simulink model "Project1_SPXMMA001"  (R2021a)
settings: Solver=ode1  StartTime=0.0  StopTime=Inf  RelTol=1e-3
InitFcn:
  |  TOFF_InitialValue.PRE = 12000;
  | OFF_InitialValue.PRE = 12000;
  | TON_InitialValue.PRE = 2000;
  | ON_InitialValue.PRE = 2000;
  | T2OFF_InitialValue.PRE = 11000;
  | T2ON_InitialValue.PRE = 3000;
  | T3OFF_InitialValue.PRE = 5000;
undefined symbols (not defined in the file): BOOL, DINT, slplc
libraries: simulink x7
(part 2 of 13)

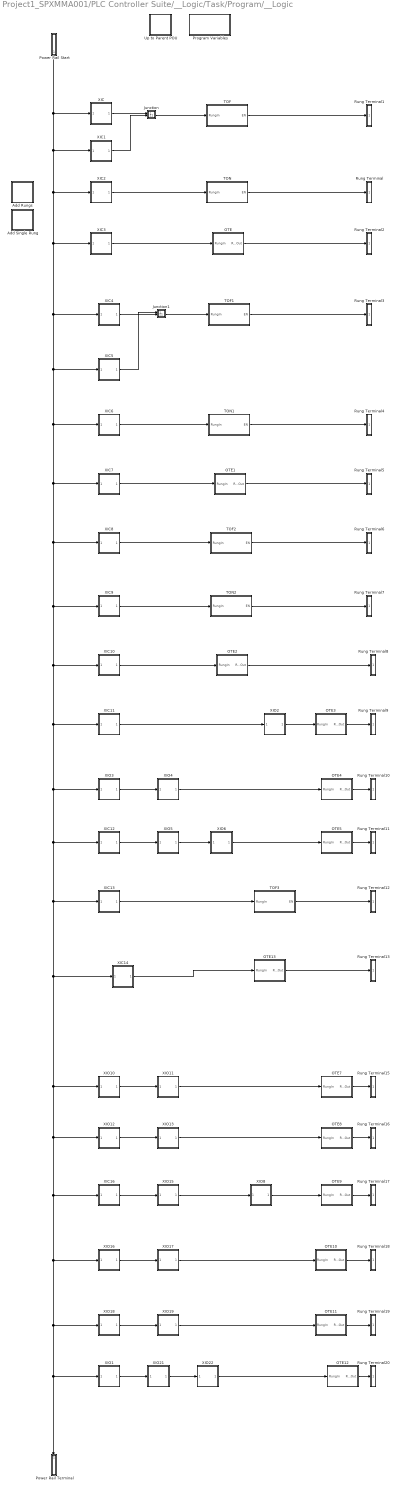
== system Project1_SPXMMA001/PLC Controller Suite/__Logic/Task/Program/__Logic ==
  Add Rungs : Subsystem  DisableCoverage=on  TreatAsAtomicUnit=on  mask{PLCRungNumberToAdd=2, PLCBlockType=AddRungs}
      mask prompts: PLCRungNumberToAdd "Rung Number:"
      mask Help: web([docroot '/plccoder/ref/addrungs' '.html']);
      mask DialogControl PLCAddRungs Prompt: Add Rungs
      mask DialogControl PLCRungAddButton Prompt: Add
      mask DialogControl PLCRungAddButton Callback: slplc.callbacks.addLadderRungs(gcb);
      mask Display: disp(sprintf(['Add' newline 'Rungs']));
  Add Single Rung : Subsystem  DisableCoverage=on  TreatAsAtomicUnit=on  mask{PLCRungNumberToAdd=1, PLCBlockType=AddSingleRung}
      settings: OpenFcn=slplc.callbacks.addLadderRungs(gcb);
      mask Help: web([docroot '/plccoder/ref/addsinglerung' '.html']);
      mask DialogControl PLCAddRung Prompt: Add Single Rung
      mask Display: disp(sprintf(['Add' newline '1 Rung']));
  Junction : Subsystem  Priority=4  DisableCoverage=on  TreatAsAtomicUnit=on  mask{PLCBlockType=Junction, PLCPOUType=BranchJunction}
      mask Help: web([docroot '/plccoder/ref/junction' '.html']);
      mask DialogControl PLCBlockTitle Prompt: Rung Merge Point
      mask DialogControl PLCBlockDesc Prompt: This is the ladder diagram rung merge point.
  Junction1 : Subsystem  Priority=15  DisableCoverage=on  TreatAsAtomicUnit=on  mask{PLCBlockType=Junction, PLCPOUType=BranchJunction}
      mask Help: web([docroot '/plccoder/ref/junction' '.html']);
      mask DialogControl PLCBlockTitle Prompt: Rung Merge Point
      mask DialogControl PLCBlockDesc Prompt: This is the ladder diagram rung merge point.
  OTE : Subsystem  Priority=11  TreatAsAtomicUnit=on  mask{PLCOperandTag=PED1_CROSS, PLCBlockType=OTE, PLCPOUType=Coil, PLCOperandExpression=xxx_PLC_VAR_PED1_CROSS}
      mask prompts: PLCOperandTag "Operand Tag:"
      mask init:
      | slplc.callbacks.initInstruction(gcb);
      settings: AttributesFormatString=%<PLCOperandTag>
      mask Help: web([docroot '/plccoder/ref/ote' '.html']);
      mask DialogControl PLCBlockTitle Prompt: Output Energize (OTE)
  OTE1 : Subsystem  Priority=22  TreatAsAtomicUnit=on  mask{PLCOperandTag=PED2_CROSS, PLCBlockType=OTE, PLCPOUType=Coil, PLCOperandExpression=xxx_PLC_VAR_PED2_CROSS}
      mask prompts: PLCOperandTag "Operand Tag:"
      mask init:
      | slplc.callbacks.initInstruction(gcb);
      settings: AttributesFormatString=%<PLCOperandTag>
      mask Help: web([docroot '/plccoder/ref/ote' '.html']);
      mask DialogControl PLCBlockTitle Prompt: Output Energize (OTE)
  OTE10 : Subsystem  Priority=67  TreatAsAtomicUnit=on  mask{PLCOperandTag=TL1_STOP, PLCBlockType=OTE, PLCPOUType=Coil, PLCOperandExpression=xxx_PLC_VAR_TL1_STOP}
      mask prompts: PLCOperandTag "Operand Tag:"
      mask init:
      | slplc.callbacks.initInstruction(gcb);
      settings: AttributesFormatString=%<PLCOperandTag>
      mask Help: web([docroot '/plccoder/ref/ote' '.html']);
      mask DialogControl PLCBlockTitle Prompt: Output Energize (OTE)
  OTE11 : Subsystem  Priority=71  TreatAsAtomicUnit=on  mask{PLCOperandTag=TL1_SO, PLCBlockType=OTE, PLCPOUType=Coil, PLCOperandExpression=xxx_PLC_VAR_TL1_SO}
      mask prompts: PLCOperandTag "Operand Tag:"
      mask init:
      | slplc.callbacks.initInstruction(gcb);
      settings: AttributesFormatString=%<PLCOperandTag>
      mask Help: web([docroot '/plccoder/ref/ote' '.html']);
      mask DialogControl PLCBlockTitle Prompt: Output Energize (OTE)
  OTE12 : Subsystem  Priority=76  TreatAsAtomicUnit=on  mask{PLCOperandTag=TL1_RO, PLCBlockType=OTE, PLCPOUType=Coil, PLCOperandExpression=xxx_PLC_VAR_TL1_RO}
      mask prompts: PLCOperandTag "Operand Tag:"
      mask init:
      | slplc.callbacks.initInstruction(gcb);
      settings: AttributesFormatString=%<PLCOperandTag>
      mask Help: web([docroot '/plccoder/ref/ote' '.html']);
      mask DialogControl PLCBlockTitle Prompt: Output Energize (OTE)
  OTE13 : Subsystem  Priority=50  TreatAsAtomicUnit=on  mask{PLCOperandTag=ZONE2_SENSOR, PLCBlockType=OTE, PLCPOUType=Coil, PLCOperandExpression=xxx_PLC_VAR_ZONE2_SENSOR}
      mask prompts: PLCOperandTag "Operand Tag:"
      mask init:
      | slplc.callbacks.initInstruction(gcb);
      settings: AttributesFormatString=%<PLCOperandTag>
      mask Help: web([docroot '/plccoder/ref/ote' '.html']);
      mask DialogControl PLCBlockTitle Prompt: Output Energize (OTE)
  OTE2 : Subsystem  Priority=31  TreatAsAtomicUnit=on  mask{PLCOperandTag=ZONE1_SENSOR, PLCBlockType=OTE, PLCPOUType=Coil, PLCOperandExpression=xxx_PLC_VAR_ZONE1_SENSOR}
      mask prompts: PLCOperandTag "Operand Tag:"
      mask init:
      | slplc.callbacks.initInstruction(gcb);
      settings: AttributesFormatString=%<PLCOperandTag>
      mask Help: web([docroot '/plccoder/ref/ote' '.html']);
      mask DialogControl PLCBlockTitle Prompt: Output Energize (OTE)
  OTE3 : Subsystem  Priority=35  TreatAsAtomicUnit=on  mask{PLCOperandTag=TL3_RO, PLCBlockType=OTE, PLCPOUType=Coil, PLCOperandExpression=xxx_PLC_VAR_TL3_RO}
      mask prompts: PLCOperandTag "Operand Tag:"
      mask init:
      | slplc.callbacks.initInstruction(gcb);
      settings: AttributesFormatString=%<PLCOperandTag>
      mask Help: web([docroot '/plccoder/ref/ote' '.html']);
      mask DialogControl PLCBlockTitle Prompt: Output Energize (OTE)
  OTE4 : Subsystem  Priority=39  TreatAsAtomicUnit=on  mask{PLCOperandTag=TL3_STOP, PLCBlockType=OTE, PLCPOUType=Coil, PLCOperandExpression=xxx_PLC_VAR_TL3_STOP}
      mask prompts: PLCOperandTag "Operand Tag:"
      mask init:
      | slplc.callbacks.initInstruction(gcb);
      settings: AttributesFormatString=%<PLCOperandTag>
      mask Help: web([docroot '/plccoder/ref/ote' '.html']);
      mask DialogControl PLCBlockTitle Prompt: Output Energize (OTE)
  OTE5 : Subsystem  Priority=44  TreatAsAtomicUnit=on  mask{PLCOperandTag=TL3_LO, PLCBlockType=OTE, PLCPOUType=Coil, PLCOperandExpression=xxx_PLC_VAR_TL3_LO}
      mask prompts: PLCOperandTag "Operand Tag:"
      mask init:
      | slplc.callbacks.initInstruction(gcb);
      settings: AttributesFormatString=%<PLCOperandTag>
      mask Help: web([docroot '/plccoder/ref/ote' '.html']);
      mask DialogControl PLCBlockTitle Prompt: Output Energize (OTE)
  OTE7 : Subsystem  Priority=54  TreatAsAtomicUnit=on  mask{PLCOperandTag=TL2_STOP, PLCBlockType=OTE, PLCPOUType=Coil, PLCOperandExpression=xxx_PLC_VAR_TL2_STOP}
      mask prompts: PLCOperandTag "Operand Tag:"
      mask init:
      | slplc.callbacks.initInstruction(gcb);
      settings: AttributesFormatString=%<PLCOperandTag>
      mask Help: web([docroot '/plccoder/ref/ote' '.html']);
      mask DialogControl PLCBlockTitle Prompt: Output Energize (OTE)
  OTE8 : Subsystem  Priority=58  TreatAsAtomicUnit=on  mask{PLCOperandTag=TL2_LO, PLCBlockType=OTE, PLCPOUType=Coil, PLCOperandExpression=xxx_PLC_VAR_TL2_LO}
      mask prompts: PLCOperandTag "Operand Tag:"
      mask init:
      | slplc.callbacks.initInstruction(gcb);
      settings: AttributesFormatString=%<PLCOperandTag>
      mask Help: web([docroot '/plccoder/ref/ote' '.html']);
      mask DialogControl PLCBlockTitle Prompt: Output Energize (OTE)
  OTE9 : Subsystem  Priority=63  TreatAsAtomicUnit=on  mask{PLCOperandTag=TL2_SO, PLCBlockType=OTE, PLCPOUType=Coil, PLCOperandExpression=xxx_PLC_VAR_TL2_SO}
      mask prompts: PLCOperandTag "Operand Tag:"
      mask init:
      | slplc.callbacks.initInstruction(gcb);
      settings: AttributesFormatString=%<PLCOperandTag>
      mask Help: web([docroot '/plccoder/ref/ote' '.html']);
      mask DialogControl PLCBlockTitle Prompt: Output Energize (OTE)
  Power Rail Start : Subsystem  Priority=1  DisableCoverage=on  TreatAsAtomicUnit=on  mask{PLCBlockType=PowerRailStart}
      mask Help: web([docroot '/plccoder/ref/powerrailstart' '.html']);
      mask DialogControl PLCBlockTitle Prompt: Power Rail Start
      mask DialogControl PLCBlockDesc Prompt: This is the ladder diagram left power rail start block.
  Power Rail Terminal : Subsystem  DisableCoverage=on  TreatAsAtomicUnit=on  mask{PLCBlockType=PowerRailTerminal}
      mask Help: web([docroot '/plccoder/ref/powerrailterminal' '.html']);
      mask DialogControl PLCBlockTitle Prompt: Power Rail Terminal
      mask DialogControl PLCBlockDesc Prompt: This is the ladder diagram left power rail terminal block.
  Program Variables : Subsystem  Tag=ProgramVariableSS  DisableCoverage=on  TreatAsAtomicUnit=on  mask{PLCVarOFFName=OFF, PLCVarOFFScope=Local, PLCVarOFFPortType=Hidden, PLCVarOFFPortIndex=32, PLCVarOFFDataType=Bus: TIMER, PLCVarOFFSize=1, PLCVarOFFInitialValue=OFF_InitialValue, PLCVarOFFToDelete=off, PLCVarONName=ON, PLCVarONScope=Local, PLCVarONPortType=Hidden, PLCVarONPortIndex=32, PLCVarONDataType=Bus: TIMER, PLCVarONSize=1, PLCVarONInitialValue=ON_InitialValue, PLCVarONToDelete=off, PLCVarPED1Name=PED1, PLCVarPED1Scope=Local, PLCVarPED1PortType=Hidden, PLCVarPED1PortIndex=32, PLCVarPED1DataType=BOOL, PLCVarPED1Size=1, PLCVarPED1InitialValue=false, PLCVarPED1ToDelete=off, PLCVarPED2Name=PED2, PLCVarPED2Scope=Local, PLCVarPED2PortType=Hidden, PLCVarPED2PortIndex=32, PLCVarPED2DataType=boolean, PLCVarPED2Size=1, PLCVarPED2InitialValue=false, PLCVarPED2ToDelete=off, PLCVarPED_CROSSName=PED_CROSS, PLCVarPED_CROSSScope=Local, PLCVarPED_CROSSPortType=Hidden, PLCVarPED_CROSSPortIndex=32, PLCVarPED_CROSSDataType=BOOL, PLCVarPED_CROSSSize=1, PLCVarPED_CROSSInitialValue=false, PLCVarPED_CROSSToDelete=off, PLCVarT2OFFName=T2OFF, PLCVarT2OFFScope=Local, PLCVarT2OFFPortType=Hidden, PLCVarT2OFFPortIndex=32, PLCVarT2OFFDataType=Bus: TIMER, PLCVarT2OFFSize=1, PLCVarT2OFFInitialValue=T2OFF_InitialValue, PLCVarT2OFFToDelete=off, PLCVarT2ONName=T2ON, PLCVarT2ONScope=Local, PLCVarT2ONPortType=Hidden, PLCVarT2ONPortIndex=32, PLCVarT2ONDataType=Bus: TIMER, PLCVarT2ONSize=1, PLCVarT2ONInitialValue=T2ON_InitialValue, PLCVarT2ONToDelete=off, PLCVarT3OFFName=T3OFF, PLCVarT3OFFScope=Local, PLCVarT3OFFPortType=Hidden, PLCVarT3OFFPortIndex=32, PLCVarT3OFFDataType=Bus: TIMER, PLCVarT3OFFSize=1, PLCVarT3OFFInitialValue=TOF_InitialValue, PLCVarT3OFFToDelete=off, PLCVarT3ONName=T3ON, PLCVarT3ONScope=Local, PLCVarT3ONPortType=Hidden, PLCVarT3ONPortIndex=32, PLCVarT3ONDataType=Bus: TIMER, PLCVarT3ONSize=1, PLCVarT3ONInitialValue=TON_InitialValue, PLCVarT3ONToDelete=off, PLCVarTL1_NOName=TL1_NO, PLCVarTL1_NOScope=Local, PLCVarTL1_NOPortType=Hidden, PLCVarTL1_NOPortIndex=32, PLCVarTL1_NODataType=BOOL, PLCVarTL1_NOSize=1, PLCVarTL1_NOInitialValue=false, PLCVarTL1_NOToDelete=off, PLCVarTL2_NOName=TL2_NO, PLCVarTL2_NOScope=Local, PLCVarTL2_NOPortType=Hidden, PLCVarTL2_NOPortIndex=32, PLCVarTL2_NODataType=BOOL, PLCVarTL2_NOSize=1, PLCVarTL2_NOInitialValue=false, PLCVarTL2_NOToDelete=off, PLCVarTOFFName=TOFF, PLCVarTOFFScope=Local, PLCVarTOFFPortType=Hidden, PLCVarTOFFPortIndex=32, PLCVarTOFFDataType=Bus: TIMER, PLCVarTOFFSize=1, PLCVarTOFFInitialValue=TOFF_InitialValue, PLCVarTOFFToDelete=off, PLCVarTONName=TON, PLCVarTONScope=Local, PLCVarTONPortType=Hidden, PLCVarTONPortIndex=32, PLCVarTONDataType=Bus: TIMER, PLCVarTONSize=1, PLCVarTONInitialValue=TON_InitialValue, PLCVarTONToDelete=off, PLCVarZONE1_SENSORName=ZONE1_SENSOR, PLCVarZONE1_SENSORScope=Local, PLCVarZONE1_SENSORPortType=Hidden, PLCVarZONE1_SENSORPortIndex=32, PLCVarZONE1_SENSORDataType=BOOL, PLCVarZONE1_SENSORSize=1, PLCVarZONE1_SENSORInitialValue=false, PLCVarZONE1_SENSORToDelete=off, PLCVarZONE2_SENSORName=ZONE2_SENSOR, PLCVarZONE2_SENSORScope=Local, PLCVarZONE2_SENSORPortType=Hidden, PLCVarZONE2_SENSORPortIndex=32, PLCVarZONE2_SENSORDataType=BOOL, PLCVarZONE2_SENSORSize=1, PLCVarZONE2_SENSORInitialValue=false, PLCVarZONE2_SENSORToDelete=off, PLCVarPED1_1Name=PED1_1, PLCVarPED1_1Scope=External, PLCVarPED1_1PortType=Hidden, PLCVarPED1_1PortIndex=32, PLCVarPED1_1DataType=DINT, PLCVarPED1_1Size=-1, PLCVarPED1_1InitialValue=0, PLCVarPED1_1ToDelete=off, PLCVarPED1_2Name=PED1_2, PLCVarPED1_2Scope=External, PLCVarPED1_2PortType=Hidden, PLCVarPED1_2PortIndex=32, PLCVarPED1_2DataType=DINT, PLCVarPED1_2Size=-1, PLCVarPED1_2InitialValue=0, PLCVarPED1_2ToDelete=off, PLCVarPED1_CROSSName=PED1_CROSS, PLCVarPED1_CROSSScope=External, PLCVarPED1_CROSSPortType=Hidden, PLCVarPED1_CROSSPortIndex=32, PLCVarPED1_CROSSDataType=DINT, PLCVarPED1_CROSSSize=-1, PLCVarPED1_CROSSInitialValue=0, PLCVarPED1_CROSSToDelete=off, PLCVarPED2_1Name=PED2_1, PLCVarPED2_1Scope=External, PLCVarPED2_1PortType=Hidden, PLCVarPED2_1PortIndex=32, PLCVarPED2_1DataType=DINT, PLCVarPED2_1Size=-1, PLCVarPED2_1InitialValue=0, PLCVarPED2_1ToDelete=off, PLCVarPED2_2Name=PED2_2, PLCVarPED2_2Scope=External, PLCVarPED2_2PortType=Hidden, PLCVarPED2_2PortIndex=32, PLCVarPED2_2DataType=DINT, PLCVarPED2_2Size=-1, PLCVarPED2_2InitialValue=0, PLCVarPED2_2ToDelete=off, PLCVarPED2_CROSSName=PED2_CROSS, PLCVarPED2_CROSSScope=External, PLCVarPED2_CROSSPortType=Hidden, PLCVarPED2_CROSSPortIndex=32, PLCVarPED2_CROSSDataType=DINT, PLCVarPED2_CROSSSize=-1, PLCVarPED2_CROSSInitialValue=0, PLCVarPED2_CROSSToDelete=off, PLCVarTL1_ROName=TL1_RO, PLCVarTL1_ROScope=External, PLCVarTL1_ROPortType=Hidden, PLCVarTL1_ROPortIndex=32, PLCVarTL1_RODataType=DINT, PLCVarTL1_ROSize=-1, PLCVarTL1_ROInitialValue=0, PLCVarTL1_ROToDelete=off, PLCVarTL1_SOName=TL1_SO, PLCVarTL1_SOScope=External, PLCVarTL1_SOPortType=Hidden, PLCVarTL1_SOPortIndex=32, PLCVarTL1_SODataType=DINT, PLCVarTL1_SOSize=-1, PLCVarTL1_SOInitialValue=0, PLCVarTL1_SOToDelete=off, PLCVarTL1_STOPName=TL1_STOP, PLCVarTL1_STOPScope=External, PLCVarTL1_STOPPortType=Hidden, PLCVarTL1_STOPPortIndex=32, PLCVarTL1_STOPDataType=DINT, PLCVarTL1_STOPSize=-1, PLCVarTL1_STOPInitialValue=0, PLCVarTL1_STOPToDelete=off, PLCVarTL2_LOName=TL2_LO, PLCVarTL2_LOScope=External, PLCVarTL2_LOPortType=Hidden, PLCVarTL2_LOPortIndex=32, PLCVarTL2_LODataType=DINT, PLCVarTL2_LOSize=-1, PLCVarTL2_LOInitialValue=0, PLCVarTL2_LOToDelete=off, PLCVarTL2_SOName=TL2_SO, PLCVarTL2_SOScope=External, PLCVarTL2_SOPortType=Hidden, PLCVarTL2_SOPortIndex=32, PLCVarTL2_SODataType=DINT, PLCVarTL2_SOSize=-1, PLCVarTL2_SOInitialValue=0, PLCVarTL2_SOToDelete=off, PLCVarTL2_STOPName=TL2_STOP, PLCVarTL2_STOPScope=External, PLCVarTL2_STOPPortType=Hidden, PLCVarTL2_STOPPortIndex=32, PLCVarTL2_STOPDataType=DINT, PLCVarTL2_STOPSize=-1, PLCVarTL2_STOPInitialValue=0, PLCVarTL2_STOPToDelete=off, PLCVarTL3_LOName=TL3_LO, PLCVarTL3_LOScope=External, PLCVarTL3_LOPortType=Hidden, PLCVarTL3_LOPortIndex=32, PLCVarTL3_LODataType=DINT, PLCVarTL3_LOSize=-1, PLCVarTL3_LOInitialValue=0, PLCVarTL3_LOToDelete=off, PLCVarTL3_ROName=TL3_RO, PLCVarTL3_ROScope=External, PLCVarTL3_ROPortType=Hidden, PLCVarTL3_ROPortIndex=32, PLCVarTL3_RODataType=DINT, PLCVarTL3_ROSize=-1, PLCVarTL3_ROInitialValue=0, PLCVarTL3_ROToDelete=off, PLCVarTL3_STOPName=TL3_STOP, PLCVarTL3_STOPScope=External, PLCVarTL3_STOPPortType=Hidden, PLCVarTL3_STOPPortIndex=32, PLCVarTL3_STOPDataType=DINT, PLCVarTL3_STOPSize=-1, PLCVarTL3_STOPInitialValue=0, PLCVarTL3_STOPToDelete=off, PLCVarZONE1Name=ZONE1, PLCVarZONE1Scope=External, PLCVarZONE1PortType=Hidden, PLCVarZONE1PortIndex=32, PLCVarZONE1DataType=DINT, PLCVarZONE1Size=-1, PLCVarZONE1InitialValue=0, PLCVarZONE1ToDelete=off, PLCVarZONE2Name=ZONE2, PLCVarZONE2Scope=External, PLCVarZONE2PortType=Hidden, PLCVarZONE2PortIndex=32, PLCVarZONE2DataType=DINT, PLCVarZONE2Size=-1, PLCVarZONE2InitialValue=0, PLCVarZONE2ToDelete=off}
      mask init:
      | slplc.callbacks.initPOUVarSS(gcb);
      settings: OpenFcn=slplc.callbacks.openProgramVariableSS(gcb);
      mask Help: web([docroot '/plccoder/ref/programvariables' '.html']);
      mask TypeOptions PLCVarOFFScope: Local | External
      mask Callback PLCVarOFFScope: slplc.callbacks.updatePOUVarSS(gcb);
      mask TypeOptions PLCVarOFFPortType: Hidden | Inport | Outport
      mask Callback PLCVarOFFPortType: slplc.callbacks.updatePOUVarSS(gcb);
      mask TypeOptions PLCVarOFFPortIndex: 1 | 2 | 3 | 4 | 5 | 6 | 7 | 8 | 9 | 10 | 11 | 12 | 13 | 14 | 15 | 16 | 17 | 18 | 19 | 20 | 21 | 22 | 23 | 24 | 25 | 26 | 27 | 28 | 29 | 30 | 31 | 32
      mask TypeOptions PLCVarONScope: Local | External
      mask Callback PLCVarONScope: slplc.callbacks.updatePOUVarSS(gcb);
      mask TypeOptions PLCVarONPortType: Hidden | Inport | Outport
      mask Callback PLCVarONPortType: slplc.callbacks.updatePOUVarSS(gcb);
      mask TypeOptions PLCVarONPortIndex: 1 | 2 | 3 | 4 | 5 | 6 | 7 | 8 | 9 | 10 | 11 | 12 | 13 | 14 | 15 | 16 | 17 | 18 | 19 | 20 | 21 | 22 | 23 | 24 | 25 | 26 | 27 | 28 | 29 | 30 | 31 | 32
      mask TypeOptions PLCVarPED1Scope: Local | External
      mask Callback PLCVarPED1Scope: slplc.callbacks.updatePOUVarSS(gcb);
      mask TypeOptions PLCVarPED1PortType: Hidden | Inport | Outport
      mask Callback PLCVarPED1PortType: slplc.callbacks.updatePOUVarSS(gcb);
      mask TypeOptions PLCVarPED1PortIndex: 1 | 2 | 3 | 4 | 5 | 6 | 7 | 8 | 9 | 10 | 11 | 12 | 13 | 14 | 15 | 16 | 17 | 18 | 19 | 20 | 21 | 22 | 23 | 24 | 25 | 26 | 27 | 28 | 29 | 30 | 31 | 32
      mask TypeOptions PLCVarPED2Scope: Local | External
      mask Callback PLCVarPED2Scope: slplc.callbacks.updatePOUVarSS(gcb);
      mask TypeOptions PLCVarPED2PortType: Hidden | Inport | Outport
      mask Callback PLCVarPED2PortType: slplc.callbacks.updatePOUVarSS(gcb);
      mask TypeOptions PLCVarPED2PortIndex: 1 | 2 | 3 | 4 | 5 | 6 | 7 | 8 | 9 | 10 | 11 | 12 | 13 | 14 | 15 | 16 | 17 | 18 | 19 | 20 | 21 | 22 | 23 | 24 | 25 | 26 | 27 | 28 | 29 | 30 | 31 | 32
      mask TypeOptions PLCVarPED_CROSSScope: Local | External
      mask Callback PLCVarPED_CROSSScope: slplc.callbacks.updatePOUVarSS(gcb);
      mask TypeOptions PLCVarPED_CROSSPortType: Hidden | Inport | Outport
      mask Callback PLCVarPED_CROSSPortType: slplc.callbacks.updatePOUVarSS(gcb);
      mask TypeOptions PLCVarPED_CROSSPortIndex: 1 | 2 | 3 | 4 | 5 | 6 | 7 | 8 | 9 | 10 | 11 | 12 | 13 | 14 | 15 | 16 | 17 | 18 | 19 | 20 | 21 | 22 | 23 | 24 | 25 | 26 | 27 | 28 | 29 | 30 | 31 | 32
      mask TypeOptions PLCVarT2OFFScope: Local | External
      mask Callback PLCVarT2OFFScope: slplc.callbacks.updatePOUVarSS(gcb);
      mask TypeOptions PLCVarT2OFFPortType: Hidden | Inport | Outport
      mask Callback PLCVarT2OFFPortType: slplc.callbacks.updatePOUVarSS(gcb);
      mask TypeOptions PLCVarT2OFFPortIndex: 1 | 2 | 3 | 4 | 5 | 6 | 7 | 8 | 9 | 10 | 11 | 12 | 13 | 14 | 15 | 16 | 17 | 18 | 19 | 20 | 21 | 22 | 23 | 24 | 25 | 26 | 27 | 28 | 29 | 30 | 31 | 32
      mask TypeOptions PLCVarT2ONScope: Local | External
      mask Callback PLCVarT2ONScope: slplc.callbacks.updatePOUVarSS(gcb);
      mask TypeOptions PLCVarT2ONPortType: Hidden | Inport | Outport
      mask Callback PLCVarT2ONPortType: slplc.callbacks.updatePOUVarSS(gcb);
      mask TypeOptions PLCVarT2ONPortIndex: 1 | 2 | 3 | 4 | 5 | 6 | 7 | 8 | 9 | 10 | 11 | 12 | 13 | 14 | 15 | 16 | 17 | 18 | 19 | 20 | 21 | 22 | 23 | 24 | 25 | 26 | 27 | 28 | 29 | 30 | 31 | 32
      mask TypeOptions PLCVarT3OFFScope: Local | External
      mask Callback PLCVarT3OFFScope: slplc.callbacks.updatePOUVarSS(gcb);
      mask TypeOptions PLCVarT3OFFPortType: Hidden | Inport | Outport
      mask Callback PLCVarT3OFFPortType: slplc.callbacks.updatePOUVarSS(gcb);
      mask TypeOptions PLCVarT3OFFPortIndex: 1 | 2 | 3 | 4 | 5 | 6 | 7 | 8 | 9 | 10 | 11 | 12 | 13 | 14 | 15 | 16 | 17 | 18 | 19 | 20 | 21 | 22 | 23 | 24 | 25 | 26 | 27 | 28 | 29 | 30 | 31 | 32
      mask TypeOptions PLCVarT3ONScope: Local | External
      mask Callback PLCVarT3ONScope: slplc.callbacks.updatePOUVarSS(gcb);
      mask TypeOptions PLCVarT3ONPortType: Hidden | Inport | Outport
      mask Callback PLCVarT3ONPortType: slplc.callbacks.updatePOUVarSS(gcb);
      mask TypeOptions PLCVarT3ONPortIndex: 1 | 2 | 3 | 4 | 5 | 6 | 7 | 8 | 9 | 10 | 11 | 12 | 13 | 14 | 15 | 16 | 17 | 18 | 19 | 20 | 21 | 22 | 23 | 24 | 25 | 26 | 27 | 28 | 29 | 30 | 31 | 32
      mask TypeOptions PLCVarTL1_NOScope: Local | External
      mask Callback PLCVarTL1_NOScope: slplc.callbacks.updatePOUVarSS(gcb);
      mask TypeOptions PLCVarTL1_NOPortType: Hidden | Inport | Outport
      mask Callback PLCVarTL1_NOPortType: slplc.callbacks.updatePOUVarSS(gcb);
      mask TypeOptions PLCVarTL1_NOPortIndex: 1 | 2 | 3 | 4 | 5 | 6 | 7 | 8 | 9 | 10 | 11 | 12 | 13 | 14 | 15 | 16 | 17 | 18 | 19 | 20 | 21 | 22 | 23 | 24 | 25 | 26 | 27 | 28 | 29 | 30 | 31 | 32
      mask TypeOptions PLCVarTL2_NOScope: Local | External
      mask Callback PLCVarTL2_NOScope: slplc.callbacks.updatePOUVarSS(gcb);
      mask TypeOptions PLCVarTL2_NOPortType: Hidden | Inport | Outport
      mask Callback PLCVarTL2_NOPortType: slplc.callbacks.updatePOUVarSS(gcb);
      mask TypeOptions PLCVarTL2_NOPortIndex: 1 | 2 | 3 | 4 | 5 | 6 | 7 | 8 | 9 | 10 | 11 | 12 | 13 | 14 | 15 | 16 | 17 | 18 | 19 | 20 | 21 | 22 | 23 | 24 | 25 | 26 | 27 | 28 | 29 | 30 | 31 | 32
      mask TypeOptions PLCVarTOFFScope: Local | External
      mask Callback PLCVarTOFFScope: slplc.callbacks.updatePOUVarSS(gcb);
      mask TypeOptions PLCVarTOFFPortType: Hidden | Inport | Outport
      mask Callback PLCVarTOFFPortType: slplc.callbacks.updatePOUVarSS(gcb);
      mask TypeOptions PLCVarTOFFPortIndex: 1 | 2 | 3 | 4 | 5 | 6 | 7 | 8 | 9 | 10 | 11 | 12 | 13 | 14 | 15 | 16 | 17 | 18 | 19 | 20 | 21 | 22 | 23 | 24 | 25 | 26 | 27 | 28 | 29 | 30 | 31 | 32
      mask TypeOptions PLCVarTONScope: Local | External
      mask Callback PLCVarTONScope: slplc.callbacks.updatePOUVarSS(gcb);
      mask TypeOptions PLCVarTONPortType: Hidden | Inport | Outport
      mask Callback PLCVarTONPortType: slplc.callbacks.updatePOUVarSS(gcb);
      mask TypeOptions PLCVarTONPortIndex: 1 | 2 | 3 | 4 | 5 | 6 | 7 | 8 | 9 | 10 | 11 | 12 | 13 | 14 | 15 | 16 | 17 | 18 | 19 | 20 | 21 | 22 | 23 | 24 | 25 | 26 | 27 | 28 | 29 | 30 | 31 | 32
      mask TypeOptions PLCVarZONE1_SENSORScope: Local | External
      mask Callback PLCVarZONE1_SENSORScope: slplc.callbacks.updatePOUVarSS(gcb);
      mask TypeOptions PLCVarZONE1_SENSORPortType: Hidden | Inport | Outport
      mask Callback PLCVarZONE1_SENSORPortType: slplc.callbacks.updatePOUVarSS(gcb);
      mask TypeOptions PLCVarZONE1_SENSORPortIndex: 1 | 2 | 3 | 4 | 5 | 6 | 7 | 8 | 9 | 10 | 11 | 12 | 13 | 14 | 15 | 16 | 17 | 18 | 19 | 20 | 21 | 22 | 23 | 24 | 25 | 26 | 27 | 28 | 29 | 30 | 31 | 32
      mask TypeOptions PLCVarZONE2_SENSORScope: Local | External
      mask Callback PLCVarZONE2_SENSORScope: slplc.callbacks.updatePOUVarSS(gcb);
      mask TypeOptions PLCVarZONE2_SENSORPortType: Hidden | Inport | Outport
      mask Callback PLCVarZONE2_SENSORPortType: slplc.callbacks.updatePOUVarSS(gcb);
      mask TypeOptions PLCVarZONE2_SENSORPortIndex: 1 | 2 | 3 | 4 | 5 | 6 | 7 | 8 | 9 | 10 | 11 | 12 | 13 | 14 | 15 | 16 | 17 | 18 | 19 | 20 | 21 | 22 | 23 | 24 | 25 | 26 | 27 | 28 | 29 | 30 | 31 | 32
      mask TypeOptions PLCVarPED1_1Scope: Local | External
      mask Callback PLCVarPED1_1Scope: slplc.callbacks.updatePOUVarSS(gcb);
      mask TypeOptions PLCVarPED1_1PortType: Hidden | Inport | Outport
      mask Callback PLCVarPED1_1PortType: slplc.callbacks.updatePOUVarSS(gcb);
      mask TypeOptions PLCVarPED1_1PortIndex: 1 | 2 | 3 | 4 | 5 | 6 | 7 | 8 | 9 | 10 | 11 | 12 | 13 | 14 | 15 | 16 | 17 | 18 | 19 | 20 | 21 | 22 | 23 | 24 | 25 | 26 | 27 | 28 | 29 | 30 | 31 | 32
      mask TypeOptions PLCVarPED1_2Scope: Local | External
      mask Callback PLCVarPED1_2Scope: slplc.callbacks.updatePOUVarSS(gcb);
      mask TypeOptions PLCVarPED1_2PortType: Hidden | Inport | Outport
      mask Callback PLCVarPED1_2PortType: slplc.callbacks.updatePOUVarSS(gcb);
      mask TypeOptions PLCVarPED1_2PortIndex: 1 | 2 | 3 | 4 | 5 | 6 | 7 | 8 | 9 | 10 | 11 | 12 | 13 | 14 | 15 | 16 | 17 | 18 | 19 | 20 | 21 | 22 | 23 | 24 | 25 | 26 | 27 | 28 | 29 | 30 | 31 | 32
      mask TypeOptions PLCVarPED1_CROSSScope: Local | External
      mask Callback PLCVarPED1_CROSSScope: slplc.callbacks.updatePOUVarSS(gcb);
      mask TypeOptions PLCVarPED1_CROSSPortType: Hidden | Inport | Outport
      mask Callback PLCVarPED1_CROSSPortType: slplc.callbacks.updatePOUVarSS(gcb);
      mask TypeOptions PLCVarPED1_CROSSPortIndex: 1 | 2 | 3 | 4 | 5 | 6 | 7 | 8 | 9 | 10 | 11 | 12 | 13 | 14 | 15 | 16 | 17 | 18 | 19 | 20 | 21 | 22 | 23 | 24 | 25 | 26 | 27 | 28 | 29 | 30 | 31 | 32
      mask TypeOptions PLCVarPED2_1Scope: Local | External
      mask Callback PLCVarPED2_1Scope: slplc.callbacks.updatePOUVarSS(gcb);
      mask TypeOptions PLCVarPED2_1PortType: Hidden | Inport | Outport
      mask Callback PLCVarPED2_1PortType: slplc.callbacks.updatePOUVarSS(gcb);
      mask TypeOptions PLCVarPED2_1PortIndex: 1 | 2 | 3 | 4 | 5 | 6 | 7 | 8 | 9 | 10 | 11 | 12 | 13 | 14 | 15 | 16 | 17 | 18 | 19 | 20 | 21 | 22 | 23 | 24 | 25 | 26 | 27 | 28 | 29 | 30 | 31 | 32
      mask TypeOptions PLCVarPED2_2Scope: Local | External
      mask Callback PLCVarPED2_2Scope: slplc.callbacks.updatePOUVarSS(gcb);
      mask TypeOptions PLCVarPED2_2PortType: Hidden | Inport | Outport
      mask Callback PLCVarPED2_2PortType: slplc.callbacks.updatePOUVarSS(gcb);
      mask TypeOptions PLCVarPED2_2PortIndex: 1 | 2 | 3 | 4 | 5 | 6 | 7 | 8 | 9 | 10 | 11 | 12 | 13 | 14 | 15 | 16 | 17 | 18 | 19 | 20 | 21 | 22 | 23 | 24 | 25 | 26 | 27 | 28 | 29 | 30 | 31 | 32
      mask TypeOptions PLCVarPED2_CROSSScope: Local | External
      mask Callback PLCVarPED2_CROSSScope: slplc.callbacks.updatePOUVarSS(gcb);
      mask TypeOptions PLCVarPED2_CROSSPortType: Hidden | Inport | Outport
      mask Callback PLCVarPED2_CROSSPortType: slplc.callbacks.updatePOUVarSS(gcb);
      mask TypeOptions PLCVarPED2_CROSSPortIndex: 1 | 2 | 3 | 4 | 5 | 6 | 7 | 8 | 9 | 10 | 11 | 12 | 13 | 14 | 15 | 16 | 17 | 18 | 19 | 20 | 21 | 22 | 23 | 24 | 25 | 26 | 27 | 28 | 29 | 30 | 31 | 32
      mask TypeOptions PLCVarTL1_ROScope: Local | External
      mask Callback PLCVarTL1_ROScope: slplc.callbacks.updatePOUVarSS(gcb);
      mask TypeOptions PLCVarTL1_ROPortType: Hidden | Inport | Outport
      mask Callback PLCVarTL1_ROPortType: slplc.callbacks.updatePOUVarSS(gcb);
      mask TypeOptions PLCVarTL1_ROPortIndex: 1 | 2 | 3 | 4 | 5 | 6 | 7 | 8 | 9 | 10 | 11 | 12 | 13 | 14 | 15 | 16 | 17 | 18 | 19 | 20 | 21 | 22 | 23 | 24 | 25 | 26 | 27 | 28 | 29 | 30 | 31 | 32
      mask TypeOptions PLCVarTL1_SOScope: Local | External
      mask Callback PLCVarTL1_SOScope: slplc.callbacks.updatePOUVarSS(gcb);
      mask TypeOptions PLCVarTL1_SOPortType: Hidden | Inport | Outport
      mask Callback PLCVarTL1_SOPortType: slplc.callbacks.updatePOUVarSS(gcb);
      mask TypeOptions PLCVarTL1_SOPortIndex: 1 | 2 | 3 | 4 | 5 | 6 | 7 | 8 | 9 | 10 | 11 | 12 | 13 | 14 | 15 | 16 | 17 | 18 | 19 | 20 | 21 | 22 | 23 | 24 | 25 | 26 | 27 | 28 | 29 | 30 | 31 | 32
      mask TypeOptions PLCVarTL1_STOPScope: Local | External
      mask Callback PLCVarTL1_STOPScope: slplc.callbacks.updatePOUVarSS(gcb);
      mask TypeOptions PLCVarTL1_STOPPortType: Hidden | Inport | Outport
      mask Callback PLCVarTL1_STOPPortType: slplc.callbacks.updatePOUVarSS(gcb);
      mask TypeOptions PLCVarTL1_STOPPortIndex: 1 | 2 | 3 | 4 | 5 | 6 | 7 | 8 | 9 | 10 | 11 | 12 | 13 | 14 | 15 | 16 | 17 | 18 | 19 | 20 | 21 | 22 | 23 | 24 | 25 | 26 | 27 | 28 | 29 | 30 | 31 | 32
      mask TypeOptions PLCVarTL2_LOScope: Local | External
      mask Callback PLCVarTL2_LOScope: slplc.callbacks.updatePOUVarSS(gcb);
      mask TypeOptions PLCVarTL2_LOPortType: Hidden | Inport | Outport
      mask Callback PLCVarTL2_LOPortType: slplc.callbacks.updatePOUVarSS(gcb);
      mask TypeOptions PLCVarTL2_LOPortIndex: 1 | 2 | 3 | 4 | 5 | 6 | 7 | 8 | 9 | 10 | 11 | 12 | 13 | 14 | 15 | 16 | 17 | 18 | 19 | 20 | 21 | 22 | 23 | 24 | 25 | 26 | 27 | 28 | 29 | 30 | 31 | 32
      mask TypeOptions PLCVarTL2_SOScope: Local | External
      mask Callback PLCVarTL2_SOScope: slplc.callbacks.updatePOUVarSS(gcb);
      mask TypeOptions PLCVarTL2_SOPortType: Hidden | Inport | Outport
      mask Callback PLCVarTL2_SOPortType: slplc.callbacks.updatePOUVarSS(gcb);
      mask TypeOptions PLCVarTL2_SOPortIndex: 1 | 2 | 3 | 4 | 5 | 6 | 7 | 8 | 9 | 10 | 11 | 12 | 13 | 14 | 15 | 16 | 17 | 18 | 19 | 20 | 21 | 22 | 23 | 24 | 25 | 26 | 27 | 28 | 29 | 30 | 31 | 32
      mask TypeOptions PLCVarTL2_STOPScope: Local | External
      mask Callback PLCVarTL2_STOPScope: slplc.callbacks.updatePOUVarSS(gcb);
      mask TypeOptions PLCVarTL2_STOPPortType: Hidden | Inport | Outport
      mask Callback PLCVarTL2_STOPPortType: slplc.callbacks.updatePOUVarSS(gcb);
      mask TypeOptions PLCVarTL2_STOPPortIndex: 1 | 2 | 3 | 4 | 5 | 6 | 7 | 8 | 9 | 10 | 11 | 12 | 13 | 14 | 15 | 16 | 17 | 18 | 19 | 20 | 21 | 22 | 23 | 24 | 25 | 26 | 27 | 28 | 29 | 30 | 31 | 32
      mask TypeOptions PLCVarTL3_LOScope: Local | External
      mask Callback PLCVarTL3_LOScope: slplc.callbacks.updatePOUVarSS(gcb);
      mask TypeOptions PLCVarTL3_LOPortType: Hidden | Inport | Outport
      mask Callback PLCVarTL3_LOPortType: slplc.callbacks.updatePOUVarSS(gcb);
      mask TypeOptions PLCVarTL3_LOPortIndex: 1 | 2 | 3 | 4 | 5 | 6 | 7 | 8 | 9 | 10 | 11 | 12 | 13 | 14 | 15 | 16 | 17 | 18 | 19 | 20 | 21 | 22 | 23 | 24 | 25 | 26 | 27 | 28 | 29 | 30 | 31 | 32
      mask TypeOptions PLCVarTL3_ROScope: Local | External
      mask Callback PLCVarTL3_ROScope: slplc.callbacks.updatePOUVarSS(gcb);
      mask TypeOptions PLCVarTL3_ROPortType: Hidden | Inport | Outport
      mask Callback PLCVarTL3_ROPortType: slplc.callbacks.updatePOUVarSS(gcb);
      mask TypeOptions PLCVarTL3_ROPortIndex: 1 | 2 | 3 | 4 | 5 | 6 | 7 | 8 | 9 | 10 | 11 | 12 | 13 | 14 | 15 | 16 | 17 | 18 | 19 | 20 | 21 | 22 | 23 | 24 | 25 | 26 | 27 | 28 | 29 | 30 | 31 | 32
      mask TypeOptions PLCVarTL3_STOPScope: Local | External
      mask Callback PLCVarTL3_STOPScope: slplc.callbacks.updatePOUVarSS(gcb);
      mask TypeOptions PLCVarTL3_STOPPortType: Hidden | Inport | Outport
      mask Callback PLCVarTL3_STOPPortType: slplc.callbacks.updatePOUVarSS(gcb);
      mask TypeOptions PLCVarTL3_STOPPortIndex: 1 | 2 | 3 | 4 | 5 | 6 | 7 | 8 | 9 | 10 | 11 | 12 | 13 | 14 | 15 | 16 | 17 | 18 | 19 | 20 | 21 | 22 | 23 | 24 | 25 | 26 | 27 | 28 | 29 | 30 | 31 | 32
      mask TypeOptions PLCVarZONE1Scope: Local | External
      mask Callback PLCVarZONE1Scope: slplc.callbacks.updatePOUVarSS(gcb);
      mask TypeOptions PLCVarZONE1PortType: Hidden | Inport | Outport
      mask Callback PLCVarZONE1PortType: slplc.callbacks.updatePOUVarSS(gcb);
      mask TypeOptions PLCVarZONE1PortIndex: 1 | 2 | 3 | 4 | 5 | 6 | 7 | 8 | 9 | 10 | 11 | 12 | 13 | 14 | 15 | 16 | 17 | 18 | 19 | 20 | 21 | 22 | 23 | 24 | 25 | 26 | 27 | 28 | 29 | 30 | 31 | 32
      mask TypeOptions PLCVarZONE2Scope: Local | External
      mask Callback PLCVarZONE2Scope: slplc.callbacks.updatePOUVarSS(gcb);
      mask TypeOptions PLCVarZONE2PortType: Hidden | Inport | Outport
      mask Callback PLCVarZONE2PortType: slplc.callbacks.updatePOUVarSS(gcb);
      mask TypeOptions PLCVarZONE2PortIndex: 1 | 2 | 3 | 4 | 5 | 6 | 7 | 8 | 9 | 10 | 11 | 12 | 13 | 14 | 15 | 16 | 17 | 18 | 19 | 20 | 21 | 22 | 23 | 24 | 25 | 26 | 27 | 28 | 29 | 30 | 31 | 32
      mask DialogControl PLCBlockTitle Prompt: Program Variable Spreadsheet
      mask DialogControl PLCVarListHeaderName Prompt: Name
      mask DialogControl PLCVarListHeaderScope Prompt: Scope
      mask DialogControl PLCVarListHeaderDataType Prompt: Data Type
      mask DialogControl PLCVarListHeaderSize Prompt: Size
      mask DialogControl PLCVarListHeaderInitialValue Prompt: Initial Value
      mask DialogControl PLCVarListHeaderToDelete Prompt: Delete
  Rung Terminal : Subsystem  Priority=9  DisableCoverage=on  TreatAsAtomicUnit=on  mask{PLCRungTerminalIndex=2, PLCBlockType=RungTerminal}
      settings: AttributesFormatString=Rung %<PLCRungTerminalIndex>
      mask Help: web([docroot '/plccoder/ref/rungterminal' '.html']);
      mask DialogControl PLCBlockTitle Prompt: Rung Terminal
      mask DialogControl PLCBlockDescText Prompt: This is the ladder diagram rung terminal.
  Rung Terminal1 : Subsystem  Priority=6  DisableCoverage=on  TreatAsAtomicUnit=on  mask{PLCRungTerminalIndex=1, PLCBlockType=RungTerminal}
      settings: AttributesFormatString=Rung %<PLCRungTerminalIndex>
      mask Help: web([docroot '/plccoder/ref/rungterminal' '.html']);
      mask DialogControl PLCBlockTitle Prompt: Rung Terminal
      mask DialogControl PLCBlockDescText Prompt: This is the ladder diagram rung terminal.
  Rung Terminal10 : Subsystem  Priority=40  DisableCoverage=on  TreatAsAtomicUnit=on  mask{PLCRungTerminalIndex=11, PLCBlockType=RungTerminal}
      settings: AttributesFormatString=Rung %<PLCRungTerminalIndex>
      mask Help: web([docroot '/plccoder/ref/rungterminal' '.html']);
      mask DialogControl PLCBlockTitle Prompt: Rung Terminal
      mask DialogControl PLCBlockDescText Prompt: This is the ladder diagram rung terminal.
  Rung Terminal11 : Subsystem  Priority=45  DisableCoverage=on  TreatAsAtomicUnit=on  mask{PLCRungTerminalIndex=12, PLCBlockType=RungTerminal}
      settings: AttributesFormatString=Rung %<PLCRungTerminalIndex>
      mask Help: web([docroot '/plccoder/ref/rungterminal' '.html']);
      mask DialogControl PLCBlockTitle Prompt: Rung Terminal
      mask DialogControl PLCBlockDescText Prompt: This is the ladder diagram rung terminal.
  Rung Terminal12 : Subsystem  Priority=48  DisableCoverage=on  TreatAsAtomicUnit=on  mask{PLCRungTerminalIndex=13, PLCBlockType=RungTerminal}
      settings: AttributesFormatString=Rung %<PLCRungTerminalIndex>
      mask Help: web([docroot '/plccoder/ref/rungterminal' '.html']);
      mask DialogControl PLCBlockTitle Prompt: Rung Terminal
      mask DialogControl PLCBlockDescText Prompt: This is the ladder diagram rung terminal.
  Rung Terminal13 : Subsystem  Priority=51  DisableCoverage=on  TreatAsAtomicUnit=on  mask{PLCRungTerminalIndex=14, PLCBlockType=RungTerminal}
      settings: AttributesFormatString=Rung %<PLCRungTerminalIndex>
      mask Help: web([docroot '/plccoder/ref/rungterminal' '.html']);
      mask DialogControl PLCBlockTitle Prompt: Rung Terminal
      mask DialogControl PLCBlockDescText Prompt: This is the ladder diagram rung terminal.
  Rung Terminal15 : Subsystem  Priority=55  DisableCoverage=on  TreatAsAtomicUnit=on  mask{PLCRungTerminalIndex=15, PLCBlockType=RungTerminal}
      settings: AttributesFormatString=Rung %<PLCRungTerminalIndex>
      mask Help: web([docroot '/plccoder/ref/rungterminal' '.html']);
      mask DialogControl PLCBlockTitle Prompt: Rung Terminal
      mask DialogControl PLCBlockDescText Prompt: This is the ladder diagram rung terminal.
  Rung Terminal16 : Subsystem  Priority=59  DisableCoverage=on  TreatAsAtomicUnit=on  mask{PLCRungTerminalIndex=16, PLCBlockType=RungTerminal}
      settings: AttributesFormatString=Rung %<PLCRungTerminalIndex>
      mask Help: web([docroot '/plccoder/ref/rungterminal' '.html']);
      mask DialogControl PLCBlockTitle Prompt: Rung Terminal
      mask DialogControl PLCBlockDescText Prompt: This is the ladder diagram rung terminal.
  Rung Terminal17 : Subsystem  Priority=64  DisableCoverage=on  TreatAsAtomicUnit=on  mask{PLCRungTerminalIndex=17, PLCBlockType=RungTerminal}
      settings: AttributesFormatString=Rung %<PLCRungTerminalIndex>
      mask Help: web([docroot '/plccoder/ref/rungterminal' '.html']);
      mask DialogControl PLCBlockTitle Prompt: Rung Terminal
      mask DialogControl PLCBlockDescText Prompt: This is the ladder diagram rung terminal.
  Rung Terminal18 : Subsystem  Priority=68  DisableCoverage=on  TreatAsAtomicUnit=on  mask{PLCRungTerminalIndex=18, PLCBlockType=RungTerminal}
      settings: AttributesFormatString=Rung %<PLCRungTerminalIndex>
      mask Help: web([docroot '/plccoder/ref/rungterminal' '.html']);
      mask DialogControl PLCBlockTitle Prompt: Rung Terminal
      mask DialogControl PLCBlockDescText Prompt: This is the ladder diagram rung terminal.
  Rung Terminal19 : Subsystem  Priority=72  DisableCoverage=on  TreatAsAtomicUnit=on  mask{PLCRungTerminalIndex=19, PLCBlockType=RungTerminal}
      settings: AttributesFormatString=Rung %<PLCRungTerminalIndex>
      mask Help: web([docroot '/plccoder/ref/rungterminal' '.html']);
      mask DialogControl PLCBlockTitle Prompt: Rung Terminal
      mask DialogControl PLCBlockDescText Prompt: This is the ladder diagram rung terminal.
  Rung Terminal2 : Subsystem  Priority=12  DisableCoverage=on  TreatAsAtomicUnit=on  mask{PLCRungTerminalIndex=3, PLCBlockType=RungTerminal}
      settings: AttributesFormatString=Rung %<PLCRungTerminalIndex>
      mask Help: web([docroot '/plccoder/ref/rungterminal' '.html']);
      mask DialogControl PLCBlockTitle Prompt: Rung Terminal
      mask DialogControl PLCBlockDescText Prompt: This is the ladder diagram rung terminal.
  Rung Terminal20 : Subsystem  Priority=77  DisableCoverage=on  TreatAsAtomicUnit=on  mask{PLCRungTerminalIndex=20, PLCBlockType=RungTerminal}
      settings: AttributesFormatString=Rung %<PLCRungTerminalIndex>
      mask Help: web([docroot '/plccoder/ref/rungterminal' '.html']);
      mask DialogControl PLCBlockTitle Prompt: Rung Terminal
      mask DialogControl PLCBlockDescText Prompt: This is the ladder diagram rung terminal.
  Rung Terminal3 : Subsystem  Priority=17  DisableCoverage=on  TreatAsAtomicUnit=on  mask{PLCRungTerminalIndex=4, PLCBlockType=RungTerminal}
      settings: AttributesFormatString=Rung %<PLCRungTerminalIndex>
      mask Help: web([docroot '/plccoder/ref/rungterminal' '.html']);
      mask DialogControl PLCBlockTitle Prompt: Rung Terminal
      mask DialogControl PLCBlockDescText Prompt: This is the ladder diagram rung terminal.
  Rung Terminal4 : Subsystem  Priority=20  DisableCoverage=on  TreatAsAtomicUnit=on  mask{PLCRungTerminalIndex=5, PLCBlockType=RungTerminal}
      settings: AttributesFormatString=Rung %<PLCRungTerminalIndex>
      mask Help: web([docroot '/plccoder/ref/rungterminal' '.html']);
      mask DialogControl PLCBlockTitle Prompt: Rung Terminal
      mask DialogControl PLCBlockDescText Prompt: This is the ladder diagram rung terminal.
  Rung Terminal5 : Subsystem  Priority=23  DisableCoverage=on  TreatAsAtomicUnit=on  mask{PLCRungTerminalIndex=6, PLCBlockType=RungTerminal}
      settings: AttributesFormatString=Rung %<PLCRungTerminalIndex>
      mask Help: web([docroot '/plccoder/ref/rungterminal' '.html']);
      mask DialogControl PLCBlockTitle Prompt: Rung Terminal
      mask DialogControl PLCBlockDescText Prompt: This is the ladder diagram rung terminal.
  Rung Terminal6 : Subsystem  Priority=26  DisableCoverage=on  TreatAsAtomicUnit=on  mask{PLCRungTerminalIndex=7, PLCBlockType=RungTerminal}
      settings: AttributesFormatString=Rung %<PLCRungTerminalIndex>
      mask Help: web([docroot '/plccoder/ref/rungterminal' '.html']);
      mask DialogControl PLCBlockTitle Prompt: Rung Terminal
      mask DialogControl PLCBlockDescText Prompt: This is the ladder diagram rung terminal.
  Rung Terminal7 : Subsystem  Priority=29  DisableCoverage=on  TreatAsAtomicUnit=on  mask{PLCRungTerminalIndex=8, PLCBlockType=RungTerminal}
      settings: AttributesFormatString=Rung %<PLCRungTerminalIndex>
      mask Help: web([docroot '/plccoder/ref/rungterminal' '.html']);
      mask DialogControl PLCBlockTitle Prompt: Rung Terminal
      mask DialogControl PLCBlockDescText Prompt: This is the ladder diagram rung terminal.
  Rung Terminal8 : Subsystem  Priority=32  DisableCoverage=on  TreatAsAtomicUnit=on  mask{PLCRungTerminalIndex=9, PLCBlockType=RungTerminal}
      settings: AttributesFormatString=Rung %<PLCRungTerminalIndex>
      mask Help: web([docroot '/plccoder/ref/rungterminal' '.html']);
      mask DialogControl PLCBlockTitle Prompt: Rung Terminal
      mask DialogControl PLCBlockDescText Prompt: This is the ladder diagram rung terminal.
  Rung Terminal9 : Subsystem  Priority=36  DisableCoverage=on  TreatAsAtomicUnit=on  mask{PLCRungTerminalIndex=10, PLCBlockType=RungTerminal}
      settings: AttributesFormatString=Rung %<PLCRungTerminalIndex>
      mask Help: web([docroot '/plccoder/ref/rungterminal' '.html']);
      mask DialogControl PLCBlockTitle Prompt: Rung Terminal
      mask DialogControl PLCBlockDescText Prompt: This is the ladder diagram rung terminal.
  TOF : Subsystem  Priority=5  TreatAsAtomicUnit=on  mask{PLCOperandTag=TOFF, PLCTimerSampleTime=0.2, PLCBlockType=TOF, PLCPOUType=stdFB, PLCOperandAccess=ReadWrite, PLCOperandExpression=xxx_PLC_VAR_TOFF}
      mask prompts: PLCOperandTag "Timer Tag:"; PLCTimerSampleTime "Timer Sample Time:"
      mask init:
      | block = gcb;
      | maskObj = Simulink.Mask.get(block);
      | maskObj.Display = sprintf('disp([''%s'' newline newline ''%s'']);', PLCBlockType, PLCOperandTag);
      | slplc.callbacks.initInstruction(block);
      settings: AttributesFormatString=%<PLCBlockType>: %<PLCOperandTag>
      mask Help: web([docroot '/plccoder/ref/tof' '.html']);
      mask DialogControl PLCBlockTitle Prompt: Timer Off Delay (TOF)
      mask Display: disp(['TOF' newline newline 'TOFF']);
  TOF1 : Subsystem  Priority=16  TreatAsAtomicUnit=on  mask{PLCOperandTag=OFF, PLCTimerSampleTime=0.2, PLCBlockType=TOF, PLCPOUType=stdFB, PLCOperandAccess=ReadWrite, PLCOperandExpression=xxx_PLC_VAR_OFF}
      mask prompts: PLCOperandTag "Timer Tag:"; PLCTimerSampleTime "Timer Sample Time:"
      mask init:
      | block = gcb;
      | maskObj = Simulink.Mask.get(block);
      | maskObj.Display = sprintf('disp([''%s'' newline newline ''%s'']);', PLCBlockType, PLCOperandTag);
      | slplc.callbacks.initInstruction(block);
      settings: AttributesFormatString=%<PLCBlockType>: %<PLCOperandTag>
      mask Help: web([docroot '/plccoder/ref/tof' '.html']);
      mask DialogControl PLCBlockTitle Prompt: Timer Off Delay (TOF)
      mask Display: disp(['TOF' newline newline 'OFF']);
  TOF2 : Subsystem  Priority=25  TreatAsAtomicUnit=on  mask{PLCOperandTag=T2OFF, PLCTimerSampleTime=0.2, PLCBlockType=TOF, PLCPOUType=stdFB, PLCOperandAccess=ReadWrite, PLCOperandExpression=xxx_PLC_VAR_T2OFF}
      mask prompts: PLCOperandTag "Timer Tag:"; PLCTimerSampleTime "Timer Sample Time:"
      mask init:
      | block = gcb;
      | maskObj = Simulink.Mask.get(block);
      | maskObj.Display = sprintf('disp([''%s'' newline newline ''%s'']);', PLCBlockType, PLCOperandTag);
      | slplc.callbacks.initInstruction(block);
      settings: AttributesFormatString=%<PLCBlockType>: %<PLCOperandTag>
      mask Help: web([docroot '/plccoder/ref/tof' '.html']);
      mask DialogControl PLCBlockTitle Prompt: Timer Off Delay (TOF)
      mask Display: disp(['TOF' newline newline 'T2OFF']);
  TOF3 : Subsystem  Priority=47  TreatAsAtomicUnit=on  mask{PLCOperandTag=T3OFF, PLCTimerSampleTime=0.2, PLCBlockType=TOF, PLCPOUType=stdFB, PLCOperandAccess=ReadWrite, PLCOperandExpression=xxx_PLC_VAR_T3OFF}
      mask prompts: PLCOperandTag "Timer Tag:"; PLCTimerSampleTime "Timer Sample Time:"
      mask init:
      | block = gcb;
      | maskObj = Simulink.Mask.get(block);
      | maskObj.Display = sprintf('disp([''%s'' newline newline ''%s'']);', PLCBlockType, PLCOperandTag);
      | slplc.callbacks.initInstruction(block);
      settings: AttributesFormatString=%<PLCBlockType>: %<PLCOperandTag>
      mask Help: web([docroot '/plccoder/ref/tof' '.html']);
      mask DialogControl PLCBlockTitle Prompt: Timer Off Delay (TOF)
      mask Display: disp(['TOF' newline newline 'T3OFF']);
  TON : Subsystem  Priority=8  TreatAsAtomicUnit=on  mask{PLCOperandTag=TON, PLCTimerSampleTime=0.2, PLCBlockType=TON, PLCPOUType=stdFB, PLCOperandAccess=ReadWrite, PLCOperandExpression=xxx_PLC_VAR_TON}
      mask prompts: PLCOperandTag "Timer Tag:"; PLCTimerSampleTime "Timer Sample Time:"
      mask init:
      | block = gcb;
      | maskObj = Simulink.Mask.get(block);
      | maskObj.Display = sprintf('disp([''%s'' newline newline ''%s'']);', PLCBlockType, PLCOperandTag);
      | slplc.callbacks.initInstruction(block);
      settings: AttributesFormatString=%<PLCBlockType>: %<PLCOperandTag>
      mask Help: web([docroot '/plccoder/ref/ton' '.html']);
      mask DialogControl PLCBlockTitle Prompt: Timer On Delay (TON)
      mask Display: disp(['TON' newline newline 'TON']);
  TON1 : Subsystem  Priority=19  TreatAsAtomicUnit=on  mask{PLCOperandTag=ON, PLCTimerSampleTime=0.2, PLCBlockType=TON, PLCPOUType=stdFB, PLCOperandAccess=ReadWrite, PLCOperandExpression=xxx_PLC_VAR_ON}
      mask prompts: PLCOperandTag "Timer Tag:"; PLCTimerSampleTime "Timer Sample Time:"
      mask init:
      | block = gcb;
      | maskObj = Simulink.Mask.get(block);
      | maskObj.Display = sprintf('disp([''%s'' newline newline ''%s'']);', PLCBlockType, PLCOperandTag);
      | slplc.callbacks.initInstruction(block);
      settings: AttributesFormatString=%<PLCBlockType>: %<PLCOperandTag>
      mask Help: web([docroot '/plccoder/ref/ton' '.html']);
      mask DialogControl PLCBlockTitle Prompt: Timer On Delay (TON)
      mask Display: disp(['TON' newline newline 'ON']);
  TON2 : Subsystem  Priority=28  TreatAsAtomicUnit=on  mask{PLCOperandTag=T2ON, PLCTimerSampleTime=0.2, PLCBlockType=TON, PLCPOUType=stdFB, PLCOperandAccess=ReadWrite, PLCOperandExpression=xxx_PLC_VAR_T2ON}
      mask prompts: PLCOperandTag "Timer Tag:"; PLCTimerSampleTime "Timer Sample Time:"
      mask init:
      | block = gcb;
      | maskObj = Simulink.Mask.get(block);
      | maskObj.Display = sprintf('disp([''%s'' newline newline ''%s'']);', PLCBlockType, PLCOperandTag);
      | slplc.callbacks.initInstruction(block);
      settings: AttributesFormatString=%<PLCBlockType>: %<PLCOperandTag>
      mask Help: web([docroot '/plccoder/ref/ton' '.html']);
      mask DialogControl PLCBlockTitle Prompt: Timer On Delay (TON)
      mask Display: disp(['TON' newline newline 'T2ON']);
  Up to Parent POU : Subsystem  DisableCoverage=on  TreatAsAtomicUnit=on  mask{PLCBlockType=OpenParentPOU}
      settings: OpenFcn=slplc.callbacks.openParentPOUBlock(gcb);
      mask Help: web([docroot '/plccoder/ref/uptoparentpou' '.html']);
      mask DialogControl PLCBlockTitle Prompt: Add Single Rung
  XIC : Subsystem  Priority=2  TreatAsAtomicUnit=on  mask{PLCOperandTag=PED1_1, PLCBlockType=XIC, PLCPOUType=Contact, PLCOperandExpression=xxx_PLC_VAR_PED1_1}
      mask prompts: PLCOperandTag "Operand Tag:"
      mask init:
      | slplc.callbacks.initInstruction(gcb);
      settings: AttributesFormatString=%<PLCOperandTag>
      mask Help: web([docroot '/plccoder/ref/xic' '.html']);
      mask DialogControl PLCBlockTitle Prompt: Examine If Closed (XIC)
  XIC1 : Subsystem  Priority=3  TreatAsAtomicUnit=on  mask{PLCOperandTag=PED1_2, PLCBlockType=XIC, PLCPOUType=Contact, PLCOperandExpression=xxx_PLC_VAR_PED1_2}
      mask prompts: PLCOperandTag "Operand Tag:"
      mask init:
      | slplc.callbacks.initInstruction(gcb);
      settings: AttributesFormatString=%<PLCOperandTag>
      mask Help: web([docroot '/plccoder/ref/xic' '.html']);
      mask DialogControl PLCBlockTitle Prompt: Examine If Closed (XIC)
  XIC10 : Subsystem  Priority=30  TreatAsAtomicUnit=on  mask{PLCOperandTag=T2ON.DN, PLCBlockType=XIC, PLCPOUType=Contact, PLCOperandExpression=xxx_PLC_VAR_T2ON.DN}
      mask prompts: PLCOperandTag "Operand Tag:"
      mask init:
      | slplc.callbacks.initInstruction(gcb);
      settings: AttributesFormatString=%<PLCOperandTag>
      mask Help: web([docroot '/plccoder/ref/xic' '.html']);
      mask DialogControl PLCBlockTitle Prompt: Examine If Closed (XIC)
  XIC11 : Subsystem  Priority=33  TreatAsAtomicUnit=on  mask{PLCOperandTag=ZONE1_SENSOR, PLCBlockType=XIC, PLCPOUType=Contact, PLCOperandExpression=xxx_PLC_VAR_ZONE1_SENSOR}
      mask prompts: PLCOperandTag "Operand Tag:"
      mask init:
      | slplc.callbacks.initInstruction(gcb);
      settings: AttributesFormatString=%<PLCOperandTag>
      mask Help: web([docroot '/plccoder/ref/xic' '.html']);
      mask DialogControl PLCBlockTitle Prompt: Examine If Closed (XIC)
  XIC12 : Subsystem  Priority=41  TreatAsAtomicUnit=on  mask{PLCOperandTag=ZONE1_SENSOR, PLCBlockType=XIC, PLCPOUType=Contact, PLCOperandExpression=xxx_PLC_VAR_ZONE1_SENSOR}
      mask prompts: PLCOperandTag "Operand Tag:"
      mask init:
      | slplc.callbacks.initInstruction(gcb);
      settings: AttributesFormatString=%<PLCOperandTag>
      mask Help: web([docroot '/plccoder/ref/xic' '.html']);
      mask DialogControl PLCBlockTitle Prompt: Examine If Closed (XIC)
  XIC13 : Subsystem  Priority=46  TreatAsAtomicUnit=on  mask{PLCOperandTag=ZONE2, PLCBlockType=XIC, PLCPOUType=Contact, PLCOperandExpression=xxx_PLC_VAR_ZONE2}
      mask prompts: PLCOperandTag "Operand Tag:"
      mask init:
      | slplc.callbacks.initInstruction(gcb);
      settings: AttributesFormatString=%<PLCOperandTag>
      mask Help: web([docroot '/plccoder/ref/xic' '.html']);
      mask DialogControl PLCBlockTitle Prompt: Examine If Closed (XIC)
  XIC14 : Subsystem  Priority=49  TreatAsAtomicUnit=on  mask{PLCOperandTag=T3OFF.DN, PLCBlockType=XIC, PLCPOUType=Contact, PLCOperandExpression=xxx_PLC_VAR_T3OFF.DN}
      mask prompts: PLCOperandTag "Operand Tag:"
      mask init:
      | slplc.callbacks.initInstruction(gcb);
      settings: AttributesFormatString=%<PLCOperandTag>
      mask Help: web([docroot '/plccoder/ref/xic' '.html']);
      mask DialogControl PLCBlockTitle Prompt: Examine If Closed (XIC)
  XIC16 : Subsystem  Priority=60  TreatAsAtomicUnit=on  mask{PLCOperandTag=TL3_STOP, PLCBlockType=XIC, PLCPOUType=Contact, PLCOperandExpression=xxx_PLC_VAR_TL3_STOP}
      mask prompts: PLCOperandTag "Operand Tag:"
      mask init:
      | slplc.callbacks.initInstruction(gcb);
      settings: AttributesFormatString=%<PLCOperandTag>
      mask Help: web([docroot '/plccoder/ref/xic' '.html']);
      mask DialogControl PLCBlockTitle Prompt: Examine If Closed (XIC)
  XIC2 : Subsystem  Priority=7  TreatAsAtomicUnit=on  mask{PLCOperandTag=TOFF.DN, PLCBlockType=XIC, PLCPOUType=Contact, PLCOperandExpression=xxx_PLC_VAR_TOFF.DN}
      mask prompts: PLCOperandTag "Operand Tag:"
      mask init:
      | slplc.callbacks.initInstruction(gcb);
      settings: AttributesFormatString=%<PLCOperandTag>
      mask Help: web([docroot '/plccoder/ref/xic' '.html']);
      mask DialogControl PLCBlockTitle Prompt: Examine If Closed (XIC)
  XIC3 : Subsystem  Priority=10  TreatAsAtomicUnit=on  mask{PLCOperandTag=TON.DN, PLCBlockType=XIC, PLCPOUType=Contact, PLCOperandExpression=xxx_PLC_VAR_TON.DN}
      mask prompts: PLCOperandTag "Operand Tag:"
      mask init:
      | slplc.callbacks.initInstruction(gcb);
      settings: AttributesFormatString=%<PLCOperandTag>
      mask Help: web([docroot '/plccoder/ref/xic' '.html']);
      mask DialogControl PLCBlockTitle Prompt: Examine If Closed (XIC)
  XIC4 : Subsystem  Priority=13  TreatAsAtomicUnit=on  mask{PLCOperandTag=PED2_1, PLCBlockType=XIC, PLCPOUType=Contact, PLCOperandExpression=xxx_PLC_VAR_PED2_1}
      mask prompts: PLCOperandTag "Operand Tag:"
      mask init:
      | slplc.callbacks.initInstruction(gcb);
      settings: AttributesFormatString=%<PLCOperandTag>
      mask Help: web([docroot '/plccoder/ref/xic' '.html']);
      mask DialogControl PLCBlockTitle Prompt: Examine If Closed (XIC)
  XIC5 : Subsystem  Priority=14  TreatAsAtomicUnit=on  mask{PLCOperandTag=PED2_2, PLCBlockType=XIC, PLCPOUType=Contact, PLCOperandExpression=xxx_PLC_VAR_PED2_2}
      mask prompts: PLCOperandTag "Operand Tag:"
      mask init:
      | slplc.callbacks.initInstruction(gcb);
      settings: AttributesFormatString=%<PLCOperandTag>
      mask Help: web([docroot '/plccoder/ref/xic' '.html']);
      mask DialogControl PLCBlockTitle Prompt: Examine If Closed (XIC)
  XIC6 : Subsystem  Priority=18  TreatAsAtomicUnit=on  mask{PLCOperandTag=OFF.DN, PLCBlockType=XIC, PLCPOUType=Contact, PLCOperandExpression=xxx_PLC_VAR_OFF.DN}
      mask prompts: PLCOperandTag "Operand Tag:"
      mask init:
      | slplc.callbacks.initInstruction(gcb);
      settings: AttributesFormatString=%<PLCOperandTag>
      mask Help: web([docroot '/plccoder/ref/xic' '.html']);
      mask DialogControl PLCBlockTitle Prompt: Examine If Closed (XIC)
  XIC7 : Subsystem  Priority=21  TreatAsAtomicUnit=on  mask{PLCOperandTag=ON.DN, PLCBlockType=XIC, PLCPOUType=Contact, PLCOperandExpression=xxx_PLC_VAR_ON.DN}
      mask prompts: PLCOperandTag "Operand Tag:"
      mask init:
      | slplc.callbacks.initInstruction(gcb);
      settings: AttributesFormatString=%<PLCOperandTag>
      mask Help: web([docroot '/plccoder/ref/xic' '.html']);
      mask DialogControl PLCBlockTitle Prompt: Examine If Closed (XIC)
  XIC8 : Subsystem  Priority=24  TreatAsAtomicUnit=on  mask{PLCOperandTag=ZONE1, PLCBlockType=XIC, PLCPOUType=Contact, PLCOperandExpression=xxx_PLC_VAR_ZONE1}
      mask prompts: PLCOperandTag "Operand Tag:"
      mask init:
      | slplc.callbacks.initInstruction(gcb);
      settings: AttributesFormatString=%<PLCOperandTag>
      mask Help: web([docroot '/plccoder/ref/xic' '.html']);
      mask DialogControl PLCBlockTitle Prompt: Examine If Closed (XIC)
  XIC9 : Subsystem  Priority=27  TreatAsAtomicUnit=on  mask{PLCOperandTag=T2OFF.DN, PLCBlockType=XIC, PLCPOUType=Contact, PLCOperandExpression=xxx_PLC_VAR_T2OFF.DN}
      mask prompts: PLCOperandTag "Operand Tag:"
      mask init:
      | slplc.callbacks.initInstruction(gcb);
      settings: AttributesFormatString=%<PLCOperandTag>
      mask Help: web([docroot '/plccoder/ref/xic' '.html']);
      mask DialogControl PLCBlockTitle Prompt: Examine If Closed (XIC)
  XIO1 : Subsystem  Priority=73  TreatAsAtomicUnit=on  mask{PLCOperandExpression=xxx_PLC_VAR_ZONE2_SENSOR, PLCOperandTag=ZONE2_SENSOR, PLCBlockType=XIO, PLCPOUType=Contact}
      mask prompts: PLCOperandTag "Operand Tag:"
      mask init:
      | slplc.callbacks.initInstruction(gcb);
      settings: AttributesFormatString=%<PLCOperandTag>
      mask Help: web([docroot '/plccoder/ref/xio' '.html']);
      mask DialogControl PLCBlockTitle Prompt: Examine If Open (XIO)
  XIO10 : Subsystem  Priority=52  TreatAsAtomicUnit=on  mask{PLCOperandExpression=xxx_PLC_VAR_TL2_LO, PLCOperandTag=TL2_LO, PLCBlockType=XIO, PLCPOUType=Contact}
      mask prompts: PLCOperandTag "Operand Tag:"
      mask init:
      | slplc.callbacks.initInstruction(gcb);
      settings: AttributesFormatString=%<PLCOperandTag>
      mask Help: web([docroot '/plccoder/ref/xio' '.html']);
      mask DialogControl PLCBlockTitle Prompt: Examine If Open (XIO)
  XIO11 : Subsystem  Priority=53  TreatAsAtomicUnit=on  mask{PLCOperandExpression=xxx_PLC_VAR_TL2_SO, PLCOperandTag=TL2_SO, PLCBlockType=XIO, PLCPOUType=Contact}
      mask prompts: PLCOperandTag "Operand Tag:"
      mask init:
      | slplc.callbacks.initInstruction(gcb);
      settings: AttributesFormatString=%<PLCOperandTag>
      mask Help: web([docroot '/plccoder/ref/xio' '.html']);
      mask DialogControl PLCBlockTitle Prompt: Examine If Open (XIO)
  XIO12 : Subsystem  Priority=56  TreatAsAtomicUnit=on  mask{PLCOperandExpression=xxx_PLC_VAR_TL1_RO, PLCOperandTag=TL1_RO, PLCBlockType=XIO, PLCPOUType=Contact}
      mask prompts: PLCOperandTag "Operand Tag:"
      mask init:
      | slplc.callbacks.initInstruction(gcb);
      settings: AttributesFormatString=%<PLCOperandTag>
      mask Help: web([docroot '/plccoder/ref/xio' '.html']);
      mask DialogControl PLCBlockTitle Prompt: Examine If Open (XIO)
  XIO13 : Subsystem  Priority=57  TreatAsAtomicUnit=on  mask{PLCOperandExpression=xxx_PLC_VAR_PED2_CROSS, PLCOperandTag=PED2_CROSS, PLCBlockType=XIO, PLCPOUType=Contact}
      mask prompts: PLCOperandTag "Operand Tag:"
      mask init:
      | slplc.callbacks.initInstruction(gcb);
      settings: AttributesFormatString=%<PLCOperandTag>
      mask Help: web([docroot '/plccoder/ref/xio' '.html']);
      mask DialogControl PLCBlockTitle Prompt: Examine If Open (XIO)
  XIO15 : Subsystem  Priority=61  TreatAsAtomicUnit=on  mask{PLCOperandExpression=xxx_PLC_VAR_PED1_CROSS, PLCOperandTag=PED1_CROSS, PLCBlockType=XIO, PLCPOUType=Contact}
      mask prompts: PLCOperandTag "Operand Tag:"
      mask init:
      | slplc.callbacks.initInstruction(gcb);
      settings: AttributesFormatString=%<PLCOperandTag>
      mask Help: web([docroot '/plccoder/ref/xio' '.html']);
      mask DialogControl PLCBlockTitle Prompt: Examine If Open (XIO)
  XIO16 : Subsystem  Priority=65  TreatAsAtomicUnit=on  mask{PLCOperandExpression=xxx_PLC_VAR_TL1_RO, PLCOperandTag=TL1_RO, PLCBlockType=XIO, PLCPOUType=Contact}
      mask prompts: PLCOperandTag "Operand Tag:"
      mask init:
      | slplc.callbacks.initInstruction(gcb);
      settings: AttributesFormatString=%<PLCOperandTag>
      mask Help: web([docroot '/plccoder/ref/xio' '.html']);
      mask DialogControl PLCBlockTitle Prompt: Examine If Open (XIO)
  XIO17 : Subsystem  Priority=66  TreatAsAtomicUnit=on  mask{PLCOperandExpression=xxx_PLC_VAR_TL1_SO, PLCOperandTag=TL1_SO, PLCBlockType=XIO, PLCPOUType=Contact}
      mask prompts: PLCOperandTag "Operand Tag:"
      mask init:
      | slplc.callbacks.initInstruction(gcb);
      settings: AttributesFormatString=%<PLCOperandTag>
      mask Help: web([docroot '/plccoder/ref/xio' '.html']);
      mask DialogControl PLCBlockTitle Prompt: Examine If Open (XIO)
  XIO18 : Subsystem  Priority=69  TreatAsAtomicUnit=on  mask{PLCOperandExpression=xxx_PLC_VAR_PED1_CROSS, PLCOperandTag=PED1_CROSS, PLCBlockType=XIO, PLCPOUType=Contact}
      mask prompts: PLCOperandTag "Operand Tag:"
      mask init:
      | slplc.callbacks.initInstruction(gcb);
      settings: AttributesFormatString=%<PLCOperandTag>
      mask Help: web([docroot '/plccoder/ref/xio' '.html']);
      mask DialogControl PLCBlockTitle Prompt: Examine If Open (XIO)
  XIO19 : Subsystem  Priority=70  TreatAsAtomicUnit=on  mask{PLCOperandExpression=xxx_PLC_VAR_TL3_RO, PLCOperandTag=TL3_RO, PLCBlockType=XIO, PLCPOUType=Contact}
      mask prompts: PLCOperandTag "Operand Tag:"
      mask init:
      | slplc.callbacks.initInstruction(gcb);
      settings: AttributesFormatString=%<PLCOperandTag>
      mask Help: web([docroot '/plccoder/ref/xio' '.html']);
      mask DialogControl PLCBlockTitle Prompt: Examine If Open (XIO)
  XIO2 : Subsystem  Priority=34  TreatAsAtomicUnit=on  mask{PLCOperandExpression=xxx_PLC_VAR_PED2_CROSS, PLCOperandTag=PED2_CROSS, PLCBlockType=XIO, PLCPOUType=Contact}
      mask prompts: PLCOperandTag "Operand Tag:"
      mask init:
      | slplc.callbacks.initInstruction(gcb);
      settings: AttributesFormatString=%<PLCOperandTag>
      mask Help: web([docroot '/plccoder/ref/xio' '.html']);
      mask DialogControl PLCBlockTitle Prompt: Examine If Open (XIO)
  XIO21 : Subsystem  Priority=74  TreatAsAtomicUnit=on  mask{PLCOperandExpression=xxx_PLC_VAR_PED1_CROSS, PLCOperandTag=PED1_CROSS, PLCBlockType=XIO, PLCPOUType=Contact}
      mask prompts: PLCOperandTag "Operand Tag:"
      mask init:
      | slplc.callbacks.initInstruction(gcb);
      settings: AttributesFormatString=%<PLCOperandTag>
      mask Help: web([docroot '/plccoder/ref/xio' '.html']);
      mask DialogControl PLCBlockTitle Prompt: Examine If Open (XIO)
  XIO22 : Subsystem  Priority=75  TreatAsAtomicUnit=on  mask{PLCOperandExpression=xxx_PLC_VAR_PED2_CROSS, PLCOperandTag=PED2_CROSS, PLCBlockType=XIO, PLCPOUType=Contact}
      mask prompts: PLCOperandTag "Operand Tag:"
      mask init:
      | slplc.callbacks.initInstruction(gcb);
      settings: AttributesFormatString=%<PLCOperandTag>
      mask Help: web([docroot '/plccoder/ref/xio' '.html']);
      mask DialogControl PLCBlockTitle Prompt: Examine If Open (XIO)
  XIO3 : Subsystem  Priority=37  TreatAsAtomicUnit=on  mask{PLCOperandExpression=xxx_PLC_VAR_TL3_LO, PLCOperandTag=TL3_LO, PLCBlockType=XIO, PLCPOUType=Contact}
      mask prompts: PLCOperandTag "Operand Tag:"
      mask init:
      | slplc.callbacks.initInstruction(gcb);
      settings: AttributesFormatString=%<PLCOperandTag>
      mask Help: web([docroot '/plccoder/ref/xio' '.html']);
      mask DialogControl PLCBlockTitle Prompt: Examine If Open (XIO)
  XIO4 : Subsystem  Priority=38  TreatAsAtomicUnit=on  mask{PLCOperandExpression=xxx_PLC_VAR_TL3_RO, PLCOperandTag=TL3_RO, PLCBlockType=XIO, PLCPOUType=Contact}
      mask prompts: PLCOperandTag "Operand Tag:"
      mask init:
      | slplc.callbacks.initInstruction(gcb);
      settings: AttributesFormatString=%<PLCOperandTag>
      mask Help: web([docroot '/plccoder/ref/xio' '.html']);
      mask DialogControl PLCBlockTitle Prompt: Examine If Open (XIO)
  XIO5 : Subsystem  Priority=42  TreatAsAtomicUnit=on  mask{PLCOperandExpression=xxx_PLC_VAR_PED1_CROSS, PLCOperandTag=PED1_CROSS, PLCBlockType=XIO, PLCPOUType=Contact}
      mask prompts: PLCOperandTag "Operand Tag:"
      mask init:
      | slplc.callbacks.initInstruction(gcb);
      settings: AttributesFormatString=%<PLCOperandTag>
      mask Help: web([docroot '/plccoder/ref/xio' '.html']);
      mask DialogControl PLCBlockTitle Prompt: Examine If Open (XIO)
  XIO6 : Subsystem  Priority=43  TreatAsAtomicUnit=on  mask{PLCOperandExpression=xxx_PLC_VAR_PED2_CROSS, PLCOperandTag=PED2_CROSS, PLCBlockType=XIO, PLCPOUType=Contact}
      mask prompts: PLCOperandTag "Operand Tag:"
      mask init:
      | slplc.callbacks.initInstruction(gcb);
      settings: AttributesFormatString=%<PLCOperandTag>
      mask Help: web([docroot '/plccoder/ref/xio' '.html']);
      mask DialogControl PLCBlockTitle Prompt: Examine If Open (XIO)
  XIO8 : Subsystem  Priority=62  TreatAsAtomicUnit=on  mask{PLCOperandExpression=xxx_PLC_VAR_TL1_RO, PLCOperandTag=TL1_RO, PLCBlockType=XIO, PLCPOUType=Contact}
      mask prompts: PLCOperandTag "Operand Tag:"
      mask init:
      | slplc.callbacks.initInstruction(gcb);
      settings: AttributesFormatString=%<PLCOperandTag>
      mask Help: web([docroot '/plccoder/ref/xio' '.html']);
      mask DialogControl PLCBlockTitle Prompt: Examine If Open (XIO)
  wires:
  Power Rail Start/1(PowerOut) -> XIC2/1(RungIn), XIC3/1(RungIn), XIC5/1(RungIn), XIC6/1(RungIn), XIC7/1(RungIn), XIC9/1(RungIn), XIC10/1(RungIn), XIC11/1(RungIn), XIO3/1(RungIn), XIC12/1(RungIn), XIO10/1(RungIn), XIO12/1(RungIn), XIC16/1(RungIn), XIO16/1(RungIn), XIO18/1(RungIn), XIO1/1(RungIn), Power Rail Terminal/1(PowerIn), XIC14/1(RungIn), XIC13/1(RungIn), XIC8/1(RungIn), XIC4/1(RungIn), XIC1/1(RungIn), XIC/1(RungIn)
  XIC/1(RungOut) -> Junction/1(RungIn1)
  Junction/1(RungOut) -> TOF/1(RungIn)
  TOF/1(EN) -> Rung Terminal1/1(RungIn)
  XIC1/1(RungOut) -> Junction/2(RungIn2)
  XIC2/1(RungOut) -> TON/1(RungIn)
  TON/1(EN) -> Rung Terminal/1(RungIn)
  XIC3/1(RungOut) -> OTE/1(RungIn)
  OTE/1(RungOut) -> Rung Terminal2/1(RungIn)
  XIC4/1(RungOut) -> Junction1/2(RungIn2)
  Junction1/1(RungOut) -> TOF1/1(RungIn)
  TOF1/1(EN) -> Rung Terminal3/1(RungIn)
  XIC5/1(RungOut) -> Junction1/1(RungIn1)
  XIC6/1(RungOut) -> TON1/1(RungIn)
  TON1/1(EN) -> Rung Terminal4/1(RungIn)
  XIC7/1(RungOut) -> OTE1/1(RungIn)
  OTE1/1(RungOut) -> Rung Terminal5/1(RungIn)
  XIC8/1(RungOut) -> TOF2/1(RungIn)
  TOF2/1(EN) -> Rung Terminal6/1(RungIn)
  XIC9/1(RungOut) -> TON2/1(RungIn)
  TON2/1(EN) -> Rung Terminal7/1(RungIn)
  XIC10/1(RungOut) -> OTE2/1(RungIn)
  OTE2/1(RungOut) -> Rung Terminal8/1(RungIn)
  XIO2/1(RungOut) -> OTE3/1(RungIn)
  OTE3/1(RungOut) -> Rung Terminal9/1(RungIn)
  XIO4/1(RungOut) -> OTE4/1(RungIn)
  XIO3/1(RungOut) -> XIO4/1(RungIn)
  OTE4/1(RungOut) -> Rung Terminal10/1(RungIn)
  OTE5/1(RungOut) -> Rung Terminal11/1(RungIn)
  XIO5/1(RungOut) -> XIO6/1(RungIn)
  XIC12/1(RungOut) -> XIO5/1(RungIn)
  XIC13/1(RungOut) -> TOF3/1(RungIn)
  TOF3/1(EN) -> Rung Terminal12/1(RungIn)
  XIC14/1(RungOut) -> OTE13/1(RungIn)
  OTE13/1(RungOut) -> Rung Terminal13/1(RungIn)
  XIO11/1(RungOut) -> OTE7/1(RungIn)
  OTE7/1(RungOut) -> Rung Terminal15/1(RungIn)
  XIO10/1(RungOut) -> XIO11/1(RungIn)
  XIO12/1(RungOut) -> XIO13/1(RungIn)
  XIO13/1(RungOut) -> OTE8/1(RungIn)
  OTE8/1(RungOut) -> Rung Terminal16/1(RungIn)
  OTE9/1(RungOut) -> Rung Terminal17/1(RungIn)
  XIO15/1(RungOut) -> XIO8/1(RungIn)
  XIC16/1(RungOut) -> XIO15/1(RungIn)
  XIO16/1(RungOut) -> XIO17/1(RungIn)
  XIO17/1(RungOut) -> OTE10/1(RungIn)
  OTE10/1(RungOut) -> Rung Terminal18/1(RungIn)
  XIO18/1(RungOut) -> XIO19/1(RungIn)
  XIO19/1(RungOut) -> OTE11/1(RungIn)
  OTE11/1(RungOut) -> Rung Terminal19/1(RungIn)
  XIO21/1(RungOut) -> XIO22/1(RungIn)
  XIO1/1(RungOut) -> XIO21/1(RungIn)
  XIO22/1(RungOut) -> OTE12/1(RungIn)
  OTE12/1(RungOut) -> Rung Terminal20/1(RungIn)
  XIO8/1(RungOut) -> OTE9/1(RungIn)
  XIO6/1(RungOut) -> OTE5/1(RungIn)
  XIC11/1(RungOut) -> XIO2/1(RungIn)
